simulink model "rtwdemo_eml_aero_radar"  (Simulink 6.0)
settings: Solver=ode5  SolverMode=SingleTasking  StartTime=0.0  StopTime=100  FixedStep=0.1  MaxStep=0.1  RelTol=1e-3  AbsTol=1e-6
PostLoadFcn:
  | rtwdemo_eml_aero_radar_data
StopFcn:
  | aero_radplot;
undefined symbols (not defined in the file or in its folder): deltat, g, Speed, tauc, tauT
libraries: simulink x2, rtwdemowidgets x1
CloseFcn:
  | h=findobj('type','figure');if ~isempty(h);close(h);end
settings Model: CovMetricSettings=d  Creator=The MathWorks Inc.  LastModifiedBy=batserve  ExtModeTrigMode=oneshot  ExtModeArmWhenConnect=off  ExtModeAutoUpdateStatusClock=off
settings DataIOCC: LimitDataPoints=off  SaveOutput=off  SaveTime=off  TimeSaveName=t_sim  SignalLoggingName=logsOut
settings OptimizationCC: InlineParams=on  EnforceIntegerDowncast=off  StateBitsets=on  DataBitsets=on  UseTempVars=on
settings DebuggingCC: CheckExecutionContextPreStartOutputMsg=on  CheckExecutionContextRuntimeOutputMsg=on  SolverPrmCheckMsg=none
settings RTWCC: TLCOptions=-p0 -aWarnNonSaturatedBlocks=0  GenerateReport=on  RTWVerbose=off  ProcessScript=grt_make_rtw_hook  LaunchReport=on
settings CodeAppCC: ForceParamTrailComments=on  MangleLength=5
settings GRTTargetCC: MatFileLogging=off

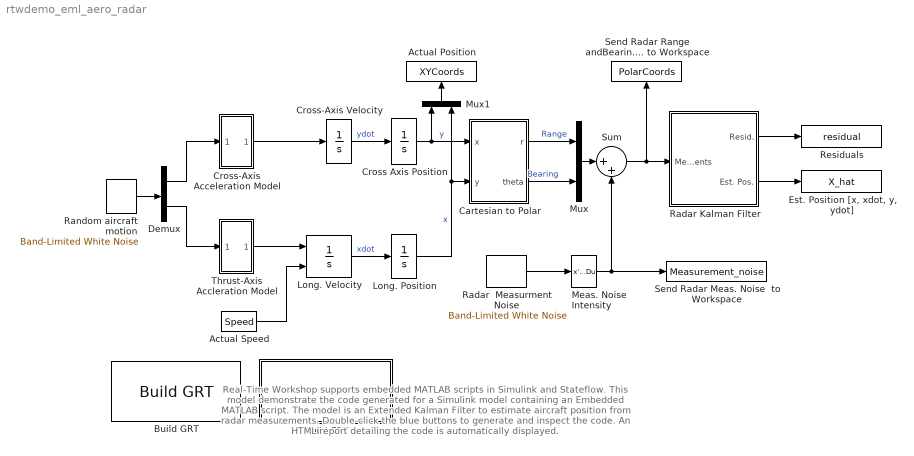
== system rtwdemo_eml_aero_radar ==
  note: Real-Time Workshop supports embedded MATLAB scripts in Simulink and Stateflow.
      | This model demonstrate the code generated for a Simulink model containing an
      | Embedded MATLAB script.  The model is an Extended Kalman Filter to estimate
      | aircraft position from radar measurements.
      |
      | Double-click the blue buttons to generate and inspect the code.  An HTML report
      | detailing the code is automatically displayed.
  Actual Position : ToWorkspace  VariableName=XYCoords  SaveFormat=Array
      settings: Orientation=up
  Actual Speed : Constant  Value=Speed
  Build ERT : Subsystem  AncestorBlock=rtwdemowidgets/Build ERT  PropExecContextAcrossSSBoundary=on  mask{attrib_overrides={}}
      mask prompts: attrib_overrides "List of attributes to preserve (cell of strings):"
      mask help: Enter the attributes of the configuration set that you want preserved. Otherwise, the default configuration script will override your current settings.
      settings: OpenFcn=|
      | model=bdroot;
      | overrides=get_param(gcb,'attrib_overrides');
      | try
      |   rtwconfiguredemo(model,'noop',false,overrides);
      |   cs = getActiveConfigSet(model);
      |   set_param(cs,'SupportNonFinite','on');
      |   rtwbuilddemomodel(model);
      | catch
      |   error(lasterr);
      | end
      mask Display:
      | disp(['Generate Code Using\n',...
      | 	  'Real-Time Workshop\n',...
      | 	  'Embedded Coder\n'...
      | 	  '(double-click)'])
  Build GRT : rtwdemowidgets/Build GRT  attrib_overrides={}
  Cartesian to Polar : Subsystem  PropExecContextAcrossSSBoundary=on
      mask Type: [x,y]->[r,theta]
      mask Description:
      | Tranformation from cartesian to polar
      | coordinates.
      | r=sqrt(x^2+y^2), theta=atan(y/x)
      mask Help: Unmask this block for more help.
      mask Display: plot(0,0,100,100,[24,20,15,20,20],[85,95,85,95,20],[80,20,95,85,95,85],[70,20,20,15,20,24],[56,56,55,52,50,46],[20,26,31,35,38,42])
  "Cross Axis Position " : Integrator
  Cross-Axis Acceleration Model : Subsystem  PropExecContextAcrossSSBoundary=on
  Cross-Axis Velocity : Integrator
  Demux : Demux  Outputs=2
  "Est. Position [x, xdot, y, ydot]" : ToWorkspace  VariableName=X_hat  SampleTime=-1  SaveFormat=Array
  Long. Position : Integrator
  Long. Velocity : Integrator  InitialConditionSource=external
  Meas. Noise Intensity : StateSpace  A=[]  B=[]  C=[]  D=K  mask(Matrix Gain){@1=[300 0; 0 .01]}
      mask prompts: @1 "Gain matrix:"
      mask help: Matrix Gain.
      mask init:
      | K = @1;
      mask Help: Multiplies input vector by entered matrix to produce output vector (y=Au).
      mask Display: disp('K')
  Mux : Mux  Inputs=2
  Mux1 : Mux  Orientation=up  Inputs=2
  Radar Kalman Filter : Subsystem  PropExecContextAcrossSSBoundary=on
  Radar  Measurment Noise : simulink/Sources/Band-Limited White Noise  Cov=[1 1]  Ts=0.1  seed=[52341 62341]
  Random aircraft motion : simulink/Sources/Band-Limited White Noise  Cov=[0.001 .001]  Ts=0.1  seed=[58413 74925]
  Residuals : ToWorkspace  VariableName=residual  SampleTime=-1  SaveFormat=Array
  Send Radar Meas. Noise  to Workspace : ToWorkspace  VariableName=Measurement_noise  SaveFormat=Array
  Send Radar Range andBearing  Angle Meas. to Workspace : ToWorkspace  VariableName=PolarCoords  SampleTime=-1  SaveFormat=Array
      settings: Orientation=up
  Sum : Sum  Inputs=|++  SaturateOnIntegerOverflow=on  InputSameDT=on
  Thrust-Axis Accleration Model : Subsystem  PropExecContextAcrossSSBoundary=on
  wires:
  Long. Position/1 -> Mux1/2, Cartesian to Polar/2(y)  "x"
  Cartesian to Polar/2(theta) -> Mux/2  "Bearing"
  Cartesian to Polar/1(r) -> Mux/1  "Range"
  Mux/1 -> Sum/1
  Sum/1 -> Radar Kalman Filter/1(Measurements), Send Radar Range andBearing  Angle Meas. to Workspace/1
  "Cross Axis Position "/1 -> Mux1/1, Cartesian to Polar/1(x)  "y"
  Cross-Axis Acceleration Model/1(out_1) -> Cross-Axis Velocity/1
  Cross-Axis Velocity/1 -> "Cross Axis Position "/1  "ydot"
  Actual Speed/1 -> Long. Velocity/2
  Long. Velocity/1 -> Long. Position/1  "xdot"
  Thrust-Axis Accleration Model/1(Accleration) -> Long. Velocity/1
  Radar Kalman Filter/1(Resid.) -> Residuals/1
  Demux/1 -> Cross-Axis Acceleration Model/1(Inport)
  Demux/2 -> Thrust-Axis Accleration Model/1(Force)
  Random aircraft motion/1 -> Demux/1
  Radar Kalman Filter/2(Est. Pos.) -> "Est. Position [x, xdot, y, ydot]"/1
  Mux1/1 -> Actual Position/1
  Radar  Measurment Noise/1 -> Meas. Noise Intensity/1
  Meas. Noise Intensity/1 -> Send Radar Meas. Noise  to Workspace/1, Sum/2

== system rtwdemo_eml_aero_radar/Build ERT ==

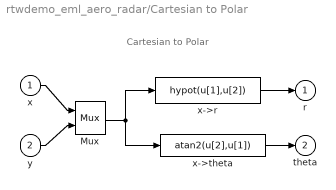
== system rtwdemo_eml_aero_radar/Cartesian to Polar ==
  note: Cartesian to Polar
  x : Inport  Port=1  LatchInput=off
  y : Inport  Port=2  LatchInput=off
  Mux : Mux  Inputs=2
  x->r : Fcn  Expr=hypot(u[1],u[2])
  x->theta : Fcn  Expr=atan2(u[2],u[1])
  r : Outport  InitialOutput=0
  theta : Outport  Port=2  InitialOutput=0
  wires:
  Mux/1 -> x->r/1, x->theta/1
  x->r/1 -> r/1
  x/1 -> Mux/1
  y/1 -> Mux/2
  x->theta/1 -> theta/1

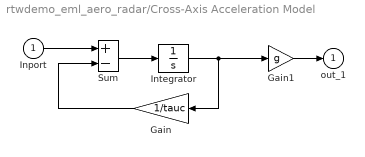
== system rtwdemo_eml_aero_radar/Cross-Axis Acceleration Model ==
  Inport : Inport  Port=1  LatchInput=off
  Gain : Gain  Orientation=left  Gain=1/tauc  SaturateOnIntegerOverflow=on
  Gain1 : Gain  Gain=g  SaturateOnIntegerOverflow=on
  Integrator : Integrator
  Sum : Sum  Inputs=+-  SaturateOnIntegerOverflow=on  InputSameDT=on
  out_1 : Outport  InitialOutput=0
  wires:
  Inport/1 -> Sum/1
  Gain/1 -> Sum/2
  Integrator/1 -> Gain1/1, Gain/1
  Sum/1 -> Integrator/1
  Gain1/1 -> out_1/1

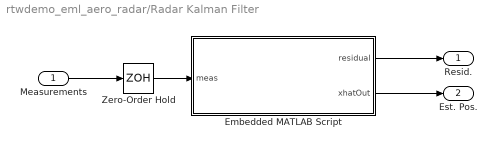
== system rtwdemo_eml_aero_radar/Radar Kalman Filter ==
  Measurements : Inport  Port=1  LatchInput=off
  Embedded MATLAB Script : Stateflow chart  PropExecContextAcrossSSBoundary=on
  Zero-Order Hold : ZeroOrderHold  SampleTime=deltat
  Resid. : Outport  InitialOutput=0
  Est. Pos. : Outport  Port=2  InitialOutput=0
  wires:
  Measurements/1 -> Zero-Order Hold/1
  Embedded MATLAB Script/1(residual) -> Resid./1
  Embedded MATLAB Script/2(xhatOut) -> Est. Pos./1
  Zero-Order Hold/1 -> Embedded MATLAB Script/1(meas)

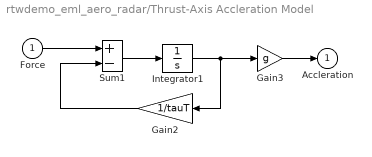
== system rtwdemo_eml_aero_radar/Thrust-Axis Accleration Model ==
  Force : Inport  Port=1  LatchInput=off
  Gain2 : Gain  Orientation=left  Gain=1/tauT  SaturateOnIntegerOverflow=on
  Gain3 : Gain  Gain=g  SaturateOnIntegerOverflow=on
  Integrator1 : Integrator
  Sum1 : Sum  Inputs=+-  SaturateOnIntegerOverflow=on  InputSameDT=on
  Accleration : Outport  InitialOutput=0
  wires:
  Force/1 -> Sum1/1
  Gain2/1 -> Sum1/2
  Integrator1/1 -> Gain3/1, Gain2/1
  Sum1/1 -> Integrator1/1
  Gain3/1 -> Accleration/1

== matlab function Radar Kalman Filter/Embedded MATLAB Script ==
  data: meas input double; residual output double; deltat parameter double size=1; xhatOut output double
function [residual, xhatOut] = AERO_EXTKALMAN(meas, deltat)
%AERO_EXTKALMAN Radar Data Processing Tracker Using an Extended Kalman Filter
%
%  This program is executed as a MATLAB function block in the 
%  aero_radmod Simulink model.  There is a file called "aero_raddat.m" that 
%  contains the data needed to run the aero_radmod model.  The estimated 
%  and actual positions are saved to the workspace and are plotted at
%  the end of the simulation by the program aero_radplot (called from the 
%  simulation automatically).
%
%  See the description in the "Extended Kalman Filter" Brochure for 
%  the equations.

%  This program was developed by Dr. Richard Gran, September 1, 1996, 
%  and modified by Paul Barnard, June 1997.
%  Copyright 1990-2002 The MathWorks, Inc.
%  $Revision: 1.1.6.3 $  $Date: 2004/04/11 00:14:59 $


% Initialization
persistent P;
persistent xhat
if isempty(P)
    xhat = [0.001; 0.01; 0.001; 400];
    P = zeros(4);
end
    
%  Radar update time deltat is inherited from workspace where it was defined by raddat.

% 1. Compute Phi, Q, and R 
Phi = [1 deltat 0 0; 0 1 0 0 ; 0 0 1 deltat; 0 0 0 1];
Q =  diag([0 .005 0 .005]);
R =  diag([300^2 0.001^2]);

% 2. Propagate the covariance matrix:
P = Phi*P*Phi' + Q;

% 3. Propagate the track estimate::
xhat = Phi*xhat;

% 4 a). Compute observation estimates:
Rangehat = sqrt(xhat(1)^2+xhat(3)^2);
Bearinghat = atan2(xhat(3),xhat(1));

% 4 b). Compute observation vector y and linearized measurement matrix M 
yhat = 	[Rangehat;
          Bearinghat];
M = [ cos(Bearinghat)          0 sin(Bearinghat)          0
   -sin(Bearinghat)/Rangehat 0 cos(Bearinghat)/Rangehat 0 ];

% 4 c).  Compute residual (Estimation Error)
residual = meas - yhat;

% 5. Compute Kalman Gain:
W = P*M'*inv(M*P*M'+ R);

% 6. Update estimate
xhat = xhat + W*residual;

% 7. Update Covariance Matrix
P = (eye(4)-W*M)*P*(eye(4)-W*M)' + W*R*W';

xhatOut = xhat;
